simulink model "motor_position_control"  (R2020b)
settings: Solver=VariableStepAuto  StartTime=0.0  StopTime=10  RelTol=1e-3
values from neighbouring files (symbols this model uses):
  b = 3.5077E-6    [motor_control_model_variables.sldd]    (also in variable_values.mat = 0.1; variables.mat = 3.5077e-06)
  J = 3.2284E-6    [motor_control_model_variables.sldd]    (also in variable_values.mat = 0.01; variables.mat = 3.2284e-06)
  K = 0.0274    [motor_control_model_variables.sldd]    (also in variable_values.mat = 0.01; variables.mat)
  Kd = -0.15    [motor_control_model_variables.sldd]    (also in variable_values.mat = 0.15; variables.mat)
  Ki = -750.0    [motor_control_model_variables.sldd]    (also in variable_values.mat = 500; variables.mat = -750)
  Kp = -20.0    [motor_control_model_variables.sldd]    (also in variable_values.mat = 20; variables.mat = -20)
  L = 2.75E-6    [motor_control_model_variables.sldd]    (also in variable_values.mat = 0.5; variables.mat = 2.75e-06)
  R = 4.0    [motor_control_model_variables.sldd]    (also in variable_values.mat = 1; variables.mat = 4)
settings Model: DataDictionary=motor_control_model_variables.sldd  Creator=DELL  LastModifiedBy=DELL
settings DataIOCC: SaveOutput=off  SaveTime=off

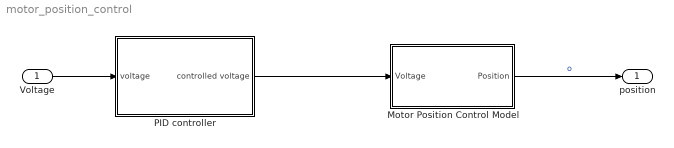
== system motor_position_control ==
  Voltage : Inport  OutDataTypeStr=double  PortDimensions=1  SampleTime=0
  Motor Position Control Model : Subsystem
  PID controller : Subsystem
  position : Outport  OutDataTypeStr=double  PortDimensions=1  SampleTime=0
  wires:
  Motor Position Control Model/1(Position) -> position/1  "o"
  Voltage/1 -> PID controller/1(voltage)
  PID controller/1(controlled voltage) -> Motor Position Control Model/1(Voltage)

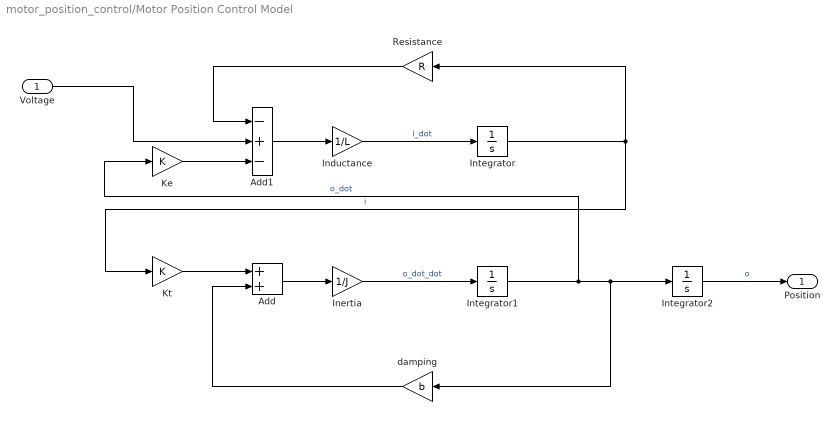
== system motor_position_control/Motor Position Control Model ==
  Voltage : Inport  OutDataTypeStr=double  PortDimensions=1  SampleTime=0
  Add : Sum
  Add1 : Sum  Inputs=-+-
  Inductance : Gain  Gain=1/L
  Inertia : Gain  Gain=1/J
  Integrator : Integrator
  Integrator1 : Integrator
  Integrator2 : Integrator
  Ke : Gain  Gain=K
  Kt : Gain  Gain=K
  Resistance : Gain  Gain=R
  damping : Gain  Gain=b
  Position : Outport  OutDataTypeStr=double  PortDimensions=1  SampleTime=0
  wires:
  Add/1 -> Inertia/1
  Integrator2/1 -> Position/1  "o"
  Kt/1 -> Add/1
  damping/1 -> Add/2
  Inductance/1 -> Integrator/1  "i_dot"
  Inertia/1 -> Integrator1/1  "o_dot_dot"
  Voltage/1 -> Add1/2
  Integrator1/1 -> Integrator2/1, damping/1, Ke/1  "o_dot"
  Resistance/1 -> Add1/1
  Add1/1 -> Inductance/1
  Integrator/1 -> Resistance/1, Kt/1  "i"
  Ke/1 -> Add1/3

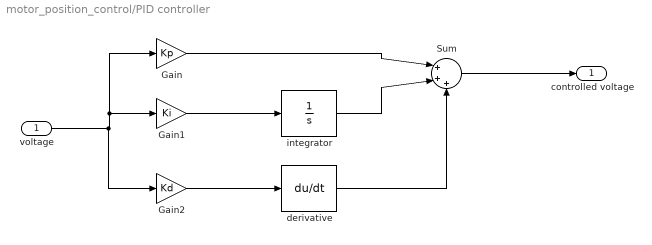
== system motor_position_control/PID controller ==
  voltage : Inport
  Gain : Gain  Gain=Kp
  Gain1 : Gain  Gain=Ki
  Gain2 : Gain  Gain=Kd
  Sum : Sum  Inputs=|+++
  derivative : Derivative
  integrator : Integrator
  controlled voltage : Outport
  wires:
  derivative/1 -> Sum/3
  Sum/1 -> controlled voltage/1
  Gain2/1 -> derivative/1
  Gain/1 -> Sum/1
  integrator/1 -> Sum/2
  voltage/1 -> Gain/1, Gain1/1, Gain2/1
  Gain1/1 -> integrator/1
